simulink model "qr"  (Simulink 8.5)
settings: Solver=ode45  StartTime=0.0  StopTime=10.0  RelTol=1e-3
InitFcn:
  | properties
settings Model: Creator=GSavaia  LastModifiedBy=GSavaia
settings DataIOCC: SignalLoggingSaveFormat=Dataset
settings OptimizationCC: ExpressionDepthLimit=128
settings DebuggingCC: UnderspecifiedInitializationDetection=Simplified  MergeDetectMultiDrivingBlocksExec=error  FcnCallInpInsideContextMsg=EnableAllAsError  StateNameClashWarn=none
settings GRTTargetCC: CombineOutputUpdateFcns=on  GRTInterface=off

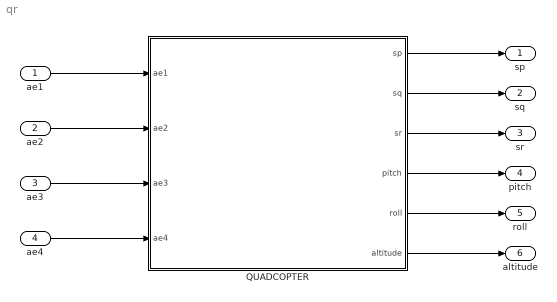
== system qr ==
  ae1 : Inport
  ae2 : Inport  Port=2
  ae3 : Inport  Port=3
  ae4 : Inport  Port=4
  QUADCOPTER : Subsystem
  sp : Outport
  sq : Outport  Port=2
  sr : Outport  Port=3
  pitch : Outport  Port=4
  roll : Outport  Port=5
  altitude : Outport  Port=6
  wires:
  ae1/1 -> QUADCOPTER/1(ae1)
  ae2/1 -> QUADCOPTER/2(ae2)
  ae3/1 -> QUADCOPTER/3(ae3)
  ae4/1 -> QUADCOPTER/4(ae4)
  QUADCOPTER/1(sp) -> sp/1
  QUADCOPTER/2(sq) -> sq/1
  QUADCOPTER/3(sr) -> sr/1
  QUADCOPTER/4(pitch) -> pitch/1
  QUADCOPTER/5(roll) -> roll/1
  QUADCOPTER/6(altitude) -> altitude/1

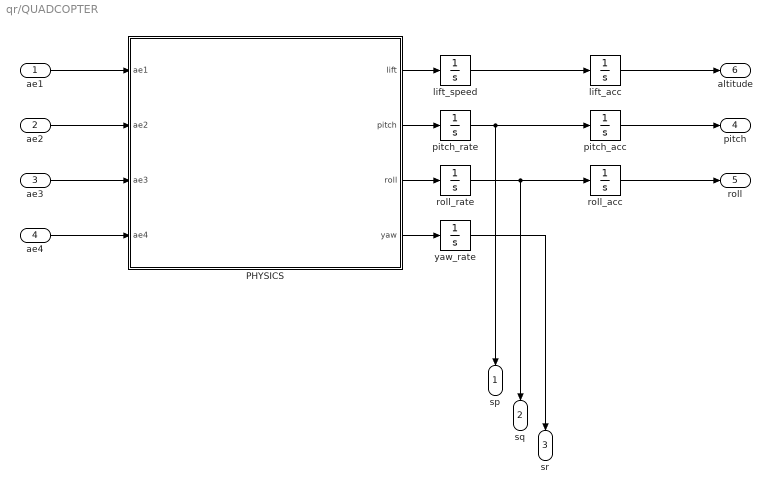
== system qr/QUADCOPTER ==
  ae1 : Inport
  ae2 : Inport  Port=2
  ae3 : Inport  Port=3
  ae4 : Inport  Port=4
  PHYSICS : MATLAB Function  TreatAsAtomicUnit=on
  lift_acc : Integrator
  lift_speed : Integrator
  pitch_acc : Integrator
  pitch_rate : Integrator
  roll_acc : Integrator
  roll_rate : Integrator
  yaw_rate : Integrator
  sp : Outport
  sq : Outport  Port=2
  sr : Outport  Port=3
  pitch : Outport  Port=4
  roll : Outport  Port=5
  altitude : Outport  Port=6
  wires:
  yaw_rate/1 -> sr/1
  roll_rate/1 -> sq/1, roll_acc/1
  ae2/1 -> PHYSICS/2(ae2)
  ae1/1 -> PHYSICS/1(ae1)
  ae3/1 -> PHYSICS/3(ae3)
  lift_acc/1 -> altitude/1
  pitch_acc/1 -> pitch/1
  lift_speed/1 -> lift_acc/1
  PHYSICS/3(roll) -> roll_rate/1
  PHYSICS/2(pitch) -> pitch_rate/1
  PHYSICS/4(yaw) -> yaw_rate/1
  PHYSICS/1(lift) -> lift_speed/1
  pitch_rate/1 -> sp/1, pitch_acc/1
  ae4/1 -> PHYSICS/4(ae4)
  roll_acc/1 -> roll/1

== matlab function QUADCOPTER/PHYSICS ==
  data: ae1 input double; lift output double; ae2 input double; ae3 input double; ae4 input double; pitch output double; roll output double; yaw output double
function [lift, pitch, roll, yaw] = motor_to_forces(ae1, ae2, ae3, ae4)

% PARAMETERS
scale_lift = 16400;
scale_pitch = 8240;
scale_roll = 8240;
scale_yaw = 16400;

lift    = 1/scale_lift*( ae1^2 + ae2^2 + ae3^2 + ae4^2 );
pitch   = 1/scale_pitch*( ae4^2 - ae2^2 );
roll    = 1/scale_roll*( ae1^2 - ae3^2 );
yaw     = 1/scale_yaw*( ae2^2 + ae4^2 - ae1^2 - ae3^2 );

end
